simulink subsystem "Plant"  (R2022a)
settings: Solver=VariableStepAuto  StartTime=0.0  StopTime=10.0  RelTol=1e-3
values from neighbouring files (symbols this model uses):
  C = [1 0 ... (first row only)    [TestDiscreteTimeSimulink.m]
  Q = Q_0*eye(N_inputs)    [TestDiscreteTimeSimulink.m]
  R = R_0*eye(N_meas)    [TestDiscreteTimeSimulink.m]
undefined symbols (not defined in the file or in its folder): C_1, C_4, R_1, R_2, R_3, R_4, Ts, x_0_2D
settings Model: Creator=tyevans  LastModifiedBy=tyevans

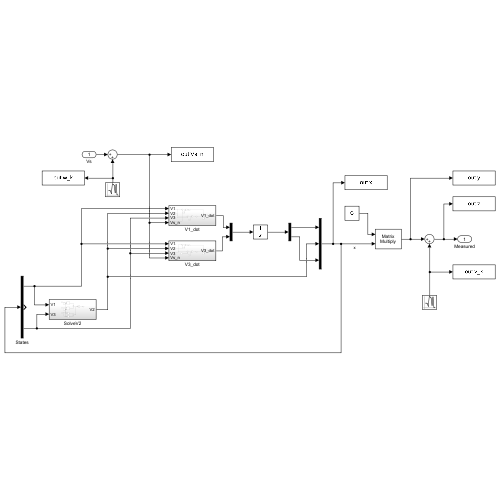
[thumbnail: Simulink's stored preview of the top-level diagram]
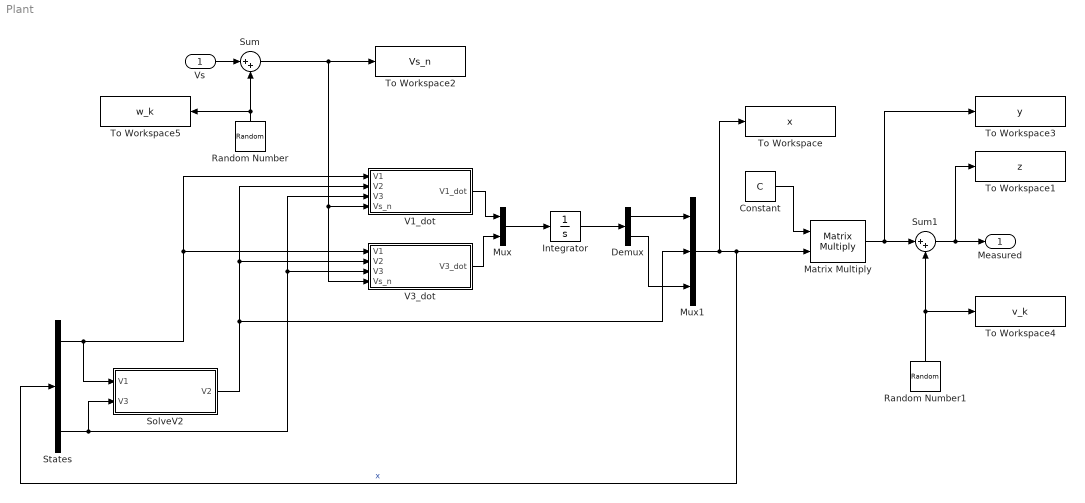
== system Plant ==
  Vs : Inport
  Constant : Constant  Value=C  VectorParams1D=off
  Demux : Demux  Outputs=2
  Integrator : Integrator  InitialCondition=x_0_2D
  Matrix Multiply : Product  Multiplication=Matrix(*)
  Mux : Mux  Inputs=2
  Mux1 : Mux  Inputs=3
  Random Number : RandomNumber  Variance=Q  SampleTime=Ts  VectorParams1D=off
  Random Number1 : RandomNumber  Variance=diag(R)  SampleTime=Ts
  SolveV2 : Subsystem
  States : Demux  Outputs=3
  Sum : Sum  Inputs=|++
  Sum1 : Sum  Inputs=|++
  To Workspace : ToWorkspace  VariableName=x  SampleTime=-1
  To Workspace1 : ToWorkspace  VariableName=z  SampleTime=-1
  To Workspace2 : ToWorkspace  VariableName=Vs_n  SampleTime=-1
  To Workspace3 : ToWorkspace  VariableName=y  SampleTime=-1
  To Workspace4 : ToWorkspace  VariableName=v_k  SampleTime=-1
  To Workspace5 : ToWorkspace  VariableName=w_k  SampleTime=-1
      settings: Save2DSignal=2-D array (concatenate along first dimension)
  V1_dot : Subsystem
  V3_dot : Subsystem
  Measured : Outport
  wires:
  Vs/1 -> Sum/1
  Random Number/1 -> To Workspace5/1, Sum/2
  Sum/1 -> V1_dot/4(Vs_n), V3_dot/4(Vs_n), To Workspace2/1
  V1_dot/1(V1_dot) -> Mux/1
  V3_dot/1(V3_dot) -> Mux/2
  Mux/1 -> Integrator/1
  Integrator/1 -> Demux/1
  Demux/1 -> Mux1/1
  Demux/2 -> Mux1/3
  Mux1/1 -> To Workspace/1, Matrix Multiply/2, States/1  "x"
  States/1 -> SolveV2/1(V1), V1_dot/1(V1), V3_dot/1(V1)
  Constant/1 -> Matrix Multiply/1
  Random Number1/1 -> Sum1/2, To Workspace4/1
  Matrix Multiply/1 -> Sum1/1, To Workspace3/1
  Sum1/1 -> To Workspace1/1, Measured/1
  SolveV2/1(V2) -> Mux1/2, V3_dot/2(V2), V1_dot/2(V2)
  States/3 -> V3_dot/3(V3), V1_dot/3(V3), SolveV2/2(V3)

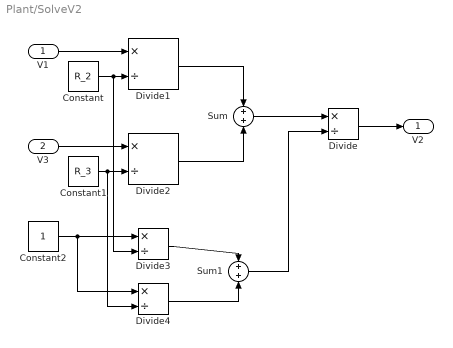
== system Plant/SolveV2 ==
  V1 : Inport
  V3 : Inport  Port=2
  Constant : Constant  Value=R_2
  Constant1 : Constant  Value=R_3
  Constant2 : Constant
  Divide{,1..4} (5 alike) : Product  Inputs=*/
  Sum : Sum
  Sum1 : Sum
  V2 : Outport
  wires:
  V1/1 -> Divide1/1
  Constant/1 -> Divide3/2, Divide1/2
  Constant1/1 -> Divide4/2, Divide2/2
  V3/1 -> Divide2/1
  Divide1/1 -> Sum/1
  Divide2/1 -> Sum/2
  Sum/1 -> Divide/1
  Divide/1 -> V2/1
  Constant2/1 -> Divide4/1, Divide3/1
  Divide3/1 -> Sum1/1
  Divide4/1 -> Sum1/2
  Sum1/1 -> Divide/2

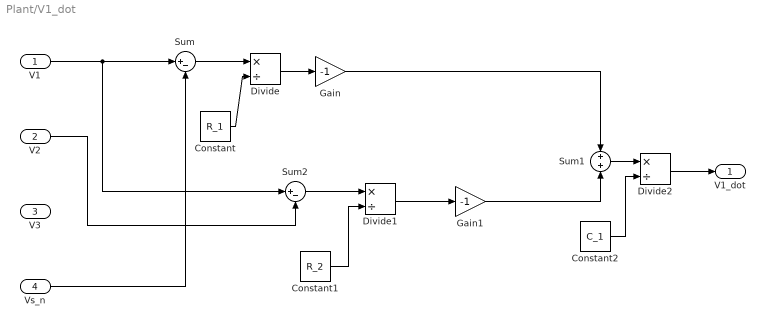
== system Plant/V1_dot ==
  V1 : Inport
  V2 : Inport  Port=2
  V3 : Inport  Port=3
  Vs_n : Inport  Port=4
  Constant : Constant  Value=R_1
  Constant1 : Constant  Value=R_2
  Constant2 : Constant  Value=C_1
  Divide : Product  Inputs=*/
  Divide1 : Product  Inputs=*/
  Divide2 : Product  Inputs=*/
  Gain : Gain  Gain=-1
  Gain1 : Gain  Gain=-1
  Sum : Sum  Inputs=|+-
  Sum1 : Sum
  Sum2 : Sum  Inputs=|+-
  V1_dot : Outport
  wires:
  V1/1 -> Sum2/1, Sum/1
  Vs_n/1 -> Sum/2
  Sum/1 -> Divide/1
  Constant/1 -> Divide/2
  Divide/1 -> Gain/1
  Gain/1 -> Sum1/1
  V2/1 -> Sum2/2
  Sum2/1 -> Divide1/1
  Constant1/1 -> Divide1/2
  Divide2/1 -> V1_dot/1
  Sum1/1 -> Divide2/1
  Divide1/1 -> Gain1/1
  Gain1/1 -> Sum1/2
  Constant2/1 -> Divide2/2

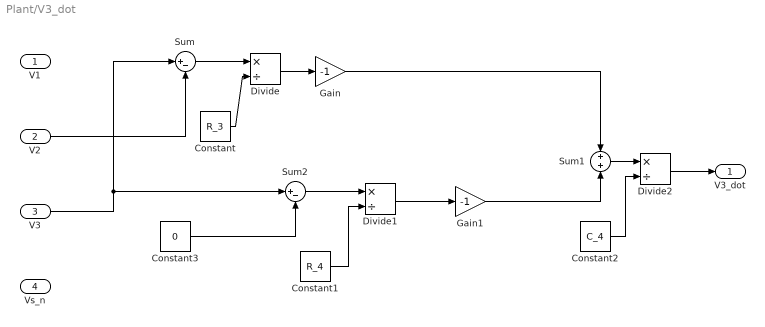
== system Plant/V3_dot ==
  V1 : Inport
  V2 : Inport  Port=2
  V3 : Inport  Port=3
  Vs_n : Inport  Port=4
  Constant : Constant  Value=R_3
  Constant1 : Constant  Value=R_4
  Constant2 : Constant  Value=C_4
  Constant3 : Constant  Value=0
  Divide : Product  Inputs=*/
  Divide1 : Product  Inputs=*/
  Divide2 : Product  Inputs=*/
  Gain : Gain  Gain=-1
  Gain1 : Gain  Gain=-1
  Sum : Sum  Inputs=|+-
  Sum1 : Sum
  Sum2 : Sum  Inputs=|+-
  V3_dot : Outport
  wires:
  Sum/1 -> Divide/1
  Constant/1 -> Divide/2
  Divide/1 -> Gain/1
  Gain/1 -> Sum1/1
  Sum2/1 -> Divide1/1
  Constant1/1 -> Divide1/2
  Divide2/1 -> V3_dot/1
  Sum1/1 -> Divide2/1
  Divide1/1 -> Gain1/1
  Gain1/1 -> Sum1/2
  Constant2/1 -> Divide2/2
  V3/1 -> Sum2/1, Sum/1
  V2/1 -> Sum/2
  Constant3/1 -> Sum2/2
